simulink model "modemodemodel1"  (R2018a)
settings: Solver=ode8  StartTime=0.0  StopTime=5  FixedStep=0.002  RelTol=1e-3
InitFcn:
  | Ao=(0.70*0.001)^2*pi/4;
  | 
  | 
  | 
  | Ar=0.38*10^-6;
  | Aor=0.1*10^-6
  | Ap=(32.50*0.001)^2*pi/4;
  | 
  | kappaaa=1.4-1.4*(Aor/Ap);
  | 
  | kappa=1.4;
  | x0=0.042;
  | P0=101325;
  | row0=1.1841;
  | T=0.005;
  | Cor=0.8;
  | 
  | Fmax=15;
  | Xmax=0.004;
  | Vmax=0.1;
  | B=0;
libraries: simulink x6, dspstat3 x1
settings Model: Creator=hiratsuka  LastModifiedBy=hiratsuka

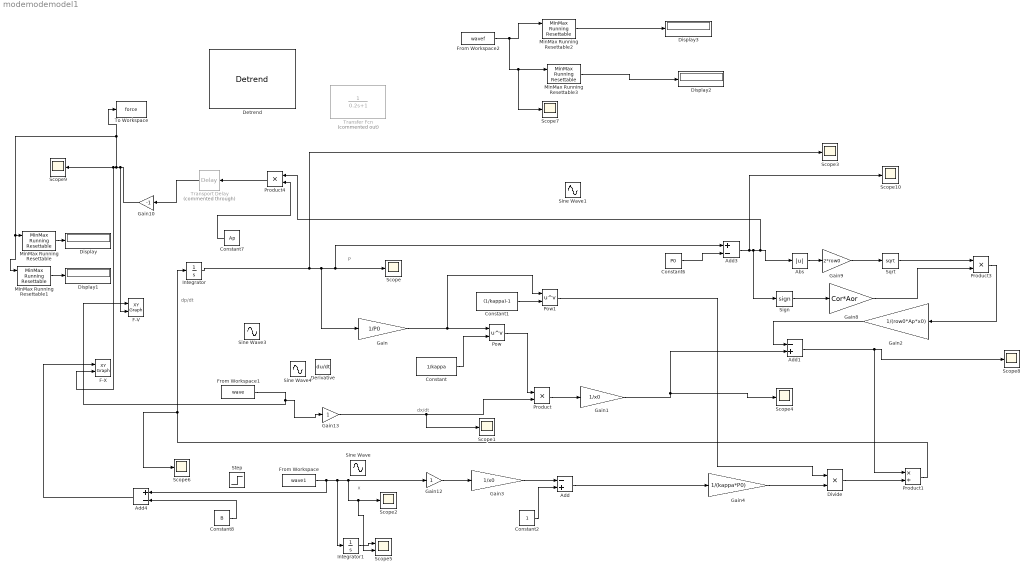
== system modemodemodel1 ==
  note: dx/dt
  note: x
  note: P
  note: dp/dt
  Abs : Abs
  Add : Sum  Inputs=-+
  Add1 : Sum  Inputs=-+
  Add3 : Sum  Inputs=+-
  Add4 : Sum  Inputs=+-
  Constant : Constant  Value=1/kappa
  Constant1 : Constant  Value=(1/kappa)-1
  Constant2 : Constant
  Constant6 : Constant  Value=P0
  Constant7 : Constant  Value=Ap
  Constant8 : Constant  Value=B
  Derivative : Derivative
  Detrend : dspstat3/Detrend
      settings: SourceProductName=DSP System Toolbox  SourceProductBaseCode=DS
  Display{,1..3} (4 alike) : Display
  Divide : Product  Inputs=**
  F-V : simulink/Sinks/XY Graph  xmin=-Vmax  xmax=Vmax  ymin=-Fmax  ymax=Fmax  st=-1
  F-X : simulink/Sinks/XY Graph  xmin=-Xmax  xmax=Xmax  ymin=-Fmax  ymax=Fmax  st=-1
  From Workspace : FromWorkspace  VariableName=wave1  SampleTime=0.002  Interpolate=off  OutputAfterFinalValue=Setting to zero
  From Workspace1 : FromWorkspace  VariableName=wave  SampleTime=0.002  Interpolate=off  OutputAfterFinalValue=Setting to zero
  From Workspace2 : FromWorkspace  VariableName=wavef  SampleTime=0.002  Interpolate=off  OutputAfterFinalValue=Setting to zero
  Gain : Gain  Gain=1/P0
  Gain1 : Gain  Gain=1/x0
  Gain10 : Gain  Gain=-1
  Gain12 : Gain
  Gain13 : Gain
  Gain2 : Gain  Gain=1/(row0*Ap*x0)
  Gain3 : Gain  Gain=1/x0
  Gain4 : Gain  Gain=1/(kappa*P0)
  Gain8 : Gain  Gain=Cor*Aor
  Gain9 : Gain  Gain=2*row0
  Integrator : Integrator  InitialCondition=101325
  Integrator1 : Integrator
  MinMax Running Resettable : simulink/Math Operations/MinMax Running Resettable  Function=max  vinit=0.0
  MinMax Running Resettable1 : simulink/Math Operations/MinMax Running Resettable  Function=min  vinit=0.0
  MinMax Running Resettable2 : simulink/Math Operations/MinMax Running Resettable  Function=max  vinit=0.0
  MinMax Running Resettable3 : simulink/Math Operations/MinMax Running Resettable  Function=min  vinit=0.0
  Pow : Math  Operator=pow  OutputSignalType=real  RndMeth=Zero  SaturateOnIntegerOverflow=on
  Pow1 : Math  Operator=pow  OutputSignalType=real  RndMeth=Zero  SaturateOnIntegerOverflow=on
  Product : Product
  Product1 : Product  Inputs=*/
  Product3 : Product
  Product4 : Product
  Scope{,1..4,6..10} (10 alike) : Scope
  Scope5 : Scope  NumInputPorts=2
  Sign : Signum
  Sine Wave : Sin  Amplitude=0.003  Bias=B  Frequency=2*pi*5  SampleTime=0
  Sine Wave1 : Sin  Bias=2  Phase=pi/2  SampleTime=0
  Sine Wave3 : Sin  Amplitude=2  Frequency=2*pi  Phase=pi/2  SampleTime=0
  Sine Wave4 : Sin  Amplitude=0.003*2*pi*5  Bias=B  Frequency=2*pi*5  Phase=pi/2  SampleTime=0
  Sqrt : Sqrt  SaturateOnIntegerOverflow=on
  Step : Step  Before=1  After=2  SampleTime=0
  To Workspace : ToWorkspace  VariableName=force  SampleTime=-1
  Transfer Fcn : TransferFcn  Commented=on  Denominator=[0.2 1]
  Transport Delay : TransportDelay  Commented=through  DelayTime=0
  wires:
  Constant/1 -> Pow/2
  Gain/1 -> Pow1/1, Pow/1
  Pow/1 -> Product/1
  Product/1 -> Gain1/1
  Constant1/1 -> Pow1/2
  Gain3/1 -> Add/1
  Constant2/1 -> Add/2
  Add/1 -> Gain4/1
  Gain4/1 -> Divide/2
  Pow1/1 -> Divide/1
  Divide/1 -> Product1/2
  Product1/1 -> Scope6/1, Integrator/1
  Sign/1 -> Gain8/1
  Constant6/1 -> Add3/2
  Integrator/1 -> Scope3/1, Gain/1, Add3/1, Scope/1
  Gain8/1 -> Product3/2
  Product3/1 -> Gain2/1
  Add1/1 -> Product1/1, Scope8/1
  Abs/1 -> Gain9/1
  Constant7/1 -> Product4/2
  Constant8/1 -> Add4/2
  Gain10/1 -> Scope9/1, F-X/2, MinMax Running Resettable1/1, MinMax Running Resettable/1, To Workspace/1, F-V/2
  Add4/1 -> F-X/1
  Gain9/1 -> Sqrt/1
  From Workspace/1 -> Integrator1/1, Gain12/1, Scope5/2, Scope2/1, Add4/1
  Gain12/1 -> Gain3/1
  From Workspace1/1 -> Gain13/1, F-V/1
  Gain2/1 -> Add1/1
  Gain13/1 -> Scope1/1, Product/2
  Gain1/1 -> Scope4/1, Add1/2
  Sqrt/1 -> Product3/1
  MinMax Running Resettable/1 -> Display/1
  MinMax Running Resettable1/1 -> Display1/1
  Add3/1 -> Scope10/1, Sign/1, Product4/1, Abs/1
  Integrator1/1 -> Scope5/1
  MinMax Running Resettable2/1 -> Display3/1
  MinMax Running Resettable3/1 -> Display2/1
  From Workspace2/1 -> Scope7/1, MinMax Running Resettable3/1, MinMax Running Resettable2/1
  Product4/1 -> Transport Delay/1
  Transport Delay/1 -> Gain10/1
